simulink model "SCARA_215_ozk_test"  (R2016a)
settings: Solver=ode1  StartTime=0.0  StopTime=100  FixedStep=0.001  RelTol=1e-3
PostLoadFcn:
  | , if any(exist('dsrtsu_mdlpostloadfcn', 'file') == [2, 3, 6]), try dsrtsu_mdlpostloadfcn('Execute', bdroot); catch fprintf('Error in PostLoadFcn (dsrtsu_mdlpostloadfcn) for model "%s":\n %s\n', bdroot, lasterr); end, end,
undefined symbols (not defined in the file): sigbuilder_block
libraries: simulink x7, simulink_extras x2
settings Model: DSRTSU_INTERNAL_RTI_VER=460  DSRTSU_INTERNAL_RTI_TYPE=rti1104  Creator=k18p800a  LastModifiedBy=Piotr
settings DataIOCC: LimitDataPoints=on  SaveFormat=Array
settings OptimizationCC: BlockReduction=off  OptimizeBlockIOStorage=off  BufferReuse=off  GlobalBufferReuse=off  ExpressionFolding=off  LocalBlockOutputs=off
settings HardwareCC: ProdBitPerPointer=32  ProdLargestAtomicFloat=None  ProdEndianess=BigEndian  ProdWordSize=32  ProdHWDeviceType=Generic->Custom  TargetIntDivRoundTo=Zero  TargetEndianess=BigEndian  TargetHWDeviceType=Generic->Custom
settings ModelReferenceCC: PropagateSignalLabelsOutOfModel=off
settings RTWCC: SystemTargetFile=rti1104.tlc  MakeCommand=make_rti  TemplateMakefile=rti1104.tmf  Description=dSPACE DS1104 Hardware Platform
settings STFCustomTargetCC: ParMdlRefBuildCompliant=on  GeneratePreprocessorConditionals=Disable all  SystemTargetFile=rti1104.tlc
settings GRTTargetCC: CompOptLevelCompliant=off  ConcurrentExecutionCompliant=off  CombineOutputUpdateFcns=off  MatFileLogging=off  CPPClassGenCompliant=off  GRTInterface=on  UseToolchainInfoCompliant=off
settings ConfigComp: CovModelRefEnable=Off

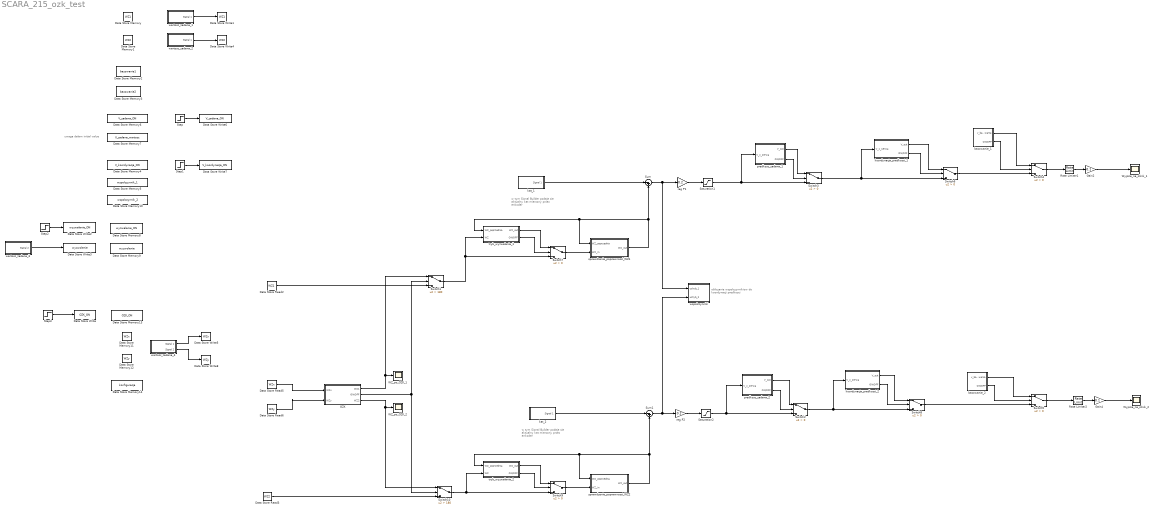
== system SCARA_215_ozk_test ==
  note: obliczanie wspolczynnikiow do
      | koordynacji predkosci
  note: w tym Signal Builder podaje
      | sie aktualny kat mierzony
      | przez enkoder
  note: w tym Signal Builder podaje
      | sie aktualny kat mierzony
      | przez enkoder
  note: uwaga dalam initial value
  Data Store Memory : DataStoreMemory  DataStoreName=WZ1  ReadBeforeWriteMsg=warning  WriteAfterWriteMsg=warning  WriteAfterReadMsg=warning  ShowAdditionalParam=off
  Data Store Memory1 : DataStoreMemory  DataStoreName=WZ2  ReadBeforeWriteMsg=warning  WriteAfterWriteMsg=warning  WriteAfterReadMsg=warning  ShowAdditionalParam=off
  Data Store Memory10 : DataStoreMemory  DataStoreName=wspolczynnik_2  ReadBeforeWriteMsg=warning  WriteAfterWriteMsg=warning  WriteAfterReadMsg=warning  ShowAdditionalParam=off
  Data Store Memory11 : DataStoreMemory  DataStoreName=WZx  ReadBeforeWriteMsg=warning  WriteAfterWriteMsg=warning  WriteAfterReadMsg=warning  ShowAdditionalParam=off
  Data Store Memory12 : DataStoreMemory  DataStoreName=WZy  ReadBeforeWriteMsg=warning  WriteAfterWriteMsg=warning  WriteAfterReadMsg=warning  ShowAdditionalParam=off
  Data Store Memory13 : DataStoreMemory  DataStoreName=OZK_ON  ReadBeforeWriteMsg=warning  WriteAfterWriteMsg=warning  WriteAfterReadMsg=warning  InitialValue=false  ShowAdditionalParam=off
  Data Store Memory14 : DataStoreMemory  DataStoreName=konfiguracja  ReadBeforeWriteMsg=warning  WriteAfterWriteMsg=warning  WriteAfterReadMsg=warning  InitialValue=false  ShowAdditionalParam=off  OutDataTypeStr=boolean
  Data Store Memory2 : DataStoreMemory  DataStoreName=bazowanie1  ReadBeforeWriteMsg=warning  WriteAfterWriteMsg=warning  WriteAfterReadMsg=warning  InitialValue=false  ShowAdditionalParam=off  OutDataTypeStr=boolean
  Data Store Memory3 : DataStoreMemory  DataStoreName=bazowanie2  ReadBeforeWriteMsg=warning  WriteAfterWriteMsg=warning  WriteAfterReadMsg=warning  InitialValue=false  ShowAdditionalParam=off  OutDataTypeStr=boolean
  Data Store Memory4 : DataStoreMemory  DataStoreName=V_koordynacja_ON  ReadBeforeWriteMsg=warning  WriteAfterWriteMsg=warning  WriteAfterReadMsg=warning  ShowAdditionalParam=off
  Data Store Memory5 : DataStoreMemory  DataStoreName=wspolczynnik_1  ReadBeforeWriteMsg=warning  WriteAfterWriteMsg=warning  WriteAfterReadMsg=warning  ShowAdditionalParam=off
  Data Store Memory6 : DataStoreMemory  DataStoreName=V_zadana_ON  ReadBeforeWriteMsg=warning  WriteAfterWriteMsg=warning  WriteAfterReadMsg=warning  ShowAdditionalParam=off
  Data Store Memory7 : DataStoreMemory  DataStoreName=V_zadana_wartosc  ReadBeforeWriteMsg=warning  WriteAfterWriteMsg=warning  WriteAfterReadMsg=warning  InitialValue=5  ShowAdditionalParam=off
  Data Store Memory8 : DataStoreMemory  DataStoreName=wyzwalanie_ON  ReadBeforeWriteMsg=warning  WriteAfterWriteMsg=warning  WriteAfterReadMsg=warning  ShowAdditionalParam=off
  Data Store Memory9 : DataStoreMemory  DataStoreName=wyzwolenie  ReadBeforeWriteMsg=warning  WriteAfterWriteMsg=warning  WriteAfterReadMsg=warning  ShowAdditionalParam=off
  Data Store Read2 : DataStoreRead  DialogController=Simulink.DDGSource  DataStoreName=WZ1
  Data Store Read3 : DataStoreRead  DialogController=Simulink.DDGSource  DataStoreName=WZ2
  Data Store Read5 : DataStoreRead  DataStoreName=WZx
  Data Store Read6 : DataStoreRead  DataStoreName=WZy
  Data Store Write : DataStoreWrite  DataStoreName=OZK_ON
  Data Store Write1 : DataStoreWrite  DataStoreName=WZ1
  Data Store Write2 : DataStoreWrite  DataStoreName=wyzwalanie_ON
  Data Store Write3 : DataStoreWrite  DataStoreName=wyzwolenie
  Data Store Write4 : DataStoreWrite  DataStoreName=WZ2
  Data Store Write5 : DataStoreWrite  DataStoreName=WZx
  Data Store Write6 : DataStoreWrite  DataStoreName=V_zadana_ON
  Data Store Write7 : DataStoreWrite  DataStoreName=V_koordynacja_ON
  Data Store Write8 : DataStoreWrite  DataStoreName=WZy
  Gain2 : Gain  Gain=0.1
  Gain4 : Gain  Gain=0.1
  OZK : Subsystem
  Rate Limiter1 : RateLimiter  RisingSlewLimit=50  FallingSlewLimit=-50  SampleTimeMode=inherited
  Rate Limiter2 : RateLimiter  RisingSlewLimit=50  FallingSlewLimit=-50  SampleTimeMode=inherited
  Saturation1 : Saturate  UpperLimit=3  LowerLimit=-3
  Saturation2 : Saturate  UpperLimit=3  LowerLimit=-3
  Step : Step  Time=50  SampleTime=0
  Step1 : Step  Time=100  SampleTime=0
  Step2 : Step  Time=100  SampleTime=0
  Step3 : Step  Time=0  SampleTime=0
  Sum : Sum  Inputs=|-+
  Sum1 : Sum  Inputs=|-+
  Switch1 : Switch  Criteria=u2 > Threshold  Threshold=180
  Switch10 : Switch  Criteria=u2 > Threshold  Threshold=180
  Switch{2..9} (8 alike) : Switch  Criteria=u2 > Threshold
  WZ_po_OZK_1 : Scope
  WZ_po_OZK_2 : Scope
  Wyjscie_na_silnik_1 : Scope
  Wyjscie_na_silnik_2 : Scope
  bazowanie_1 : Subsystem
  bazowanie_2 : Subsystem
  kat_1 : Subsystem  Tag=STV Subsys  LoadFcn=sigbuilder_block('load');  StartFcn=sigbuilder_block('start');  StopFcn=sigbuilder_block('stop');  ClipboardFcn=sigbuilder_block('clipboard');  mask(Sigbuilder block){}
      mask help: Simulink:masks:SigbuilderBlock_MD
      mask init:
      | if ~strcmp(get_param(bdroot(gcbh),'SimulationStatus'),'stopped') tuvar = sigbuilder_block('maskInit'); end
      settings: CopyFcn=sigbuilder_block('copy');  DeleteFcn=sigbuilder_block('delete');  ModelCloseFcn=sigbuilder_block('modelClose');  PreSaveFcn=sigbuilder_block('preSave');  PauseFcn=sigbuilder_block('pause');  ContinueFcn=sigbuilder_block('continue');  NameChangeFcn=sigbuilder_block('namechange');  OpenFcn=sigbuilder_block('open',[437.25 153 550.5 359.25 ]);  CloseFcn=sigbuilder_block('close');
      mask Display: plot(0, 0, 100, 100,[2, 2, 32, 32, 2], [68, 8, 8, 68, 68],[32, 2], [38, 38], [32, 19, 2],[53, 60, 44], [32, 17, 17, 2],[16, 16, 31, 31]);txt = getActiveGroup(gcbh);text(2, 100, txt,'verticalAlignment', 'top');
  kat_2 : Subsystem  Tag=STV Subsys  LoadFcn=sigbuilder_block('load');  StartFcn=sigbuilder_block('start');  StopFcn=sigbuilder_block('stop');  ClipboardFcn=sigbuilder_block('clipboard');  mask(Sigbuilder block){}
      mask help: Simulink:masks:SigbuilderBlock_MD
      mask init:
      | if ~strcmp(get_param(bdroot(gcbh),'SimulationStatus'),'stopped') tuvar = sigbuilder_block('maskInit'); end
      settings: CopyFcn=sigbuilder_block('copy');  DeleteFcn=sigbuilder_block('delete');  ModelCloseFcn=sigbuilder_block('modelClose');  PreSaveFcn=sigbuilder_block('preSave');  PauseFcn=sigbuilder_block('pause');  ContinueFcn=sigbuilder_block('continue');  NameChangeFcn=sigbuilder_block('namechange');  OpenFcn=sigbuilder_block('open',[437.25 153 550.5 359.25 ]);  CloseFcn=sigbuilder_block('close');
      mask Display: plot(0, 0, 100, 100,[2, 2, 32, 32, 2], [68, 8, 8, 68, 68],[32, 2], [38, 38], [32, 19, 2],[53, 60, 44], [32, 17, 17, 2],[16, 16, 31, 31]);txt = getActiveGroup(gcbh);text(2, 100, txt,'verticalAlignment', 'top');
  koordynacja_predkosci_1 : Subsystem
  koordynacja_predkosci_2 : Subsystem
  predkosc_zadana_1 : Subsystem
  predkosc_zadana_2 : Subsystem
  reg P1 : Gain  Gain=0.2
  reg P2 : Gain  Gain=0.2
  sprawdzenie_poprawnosci_WZ1 : Subsystem
  sprawdzenie_poprawnosci_WZ2 : Subsystem
  tryb_wyzwalania_1 : Subsystem
  tryb_wyzwalania_2 : Subsystem
  wartosc_zadana_1 : Subsystem  Tag=STV Subsys  LoadFcn=sigbuilder_block('load');  StartFcn=sigbuilder_block('start');  StopFcn=sigbuilder_block('stop');  ClipboardFcn=sigbuilder_block('clipboard');  mask(Sigbuilder block){}
      mask help: Simulink:masks:SigbuilderBlock_MD
      mask init:
      | if ~strcmp(get_param(bdroot(gcbh),'SimulationStatus'),'stopped') tuvar = sigbuilder_block('maskInit'); end
      settings: CopyFcn=sigbuilder_block('copy');  DeleteFcn=sigbuilder_block('delete');  ModelCloseFcn=sigbuilder_block('modelClose');  PreSaveFcn=sigbuilder_block('preSave');  PauseFcn=sigbuilder_block('pause');  ContinueFcn=sigbuilder_block('continue');  NameChangeFcn=sigbuilder_block('namechange');  OpenFcn=sigbuilder_block('open',[437.25 153 550.5 359.25 ]);  CloseFcn=sigbuilder_block('close');
      mask Display: plot(0, 0, 100, 100,[2, 2, 32, 32, 2], [68, 8, 8, 68, 68],[32, 2], [38, 38], [32, 19, 2],[53, 60, 44], [32, 17, 17, 2],[16, 16, 31, 31]);txt = getActiveGroup(gcbh);text(2, 100, txt,'verticalAlignment', 'top');
  wartosc_zadana_2 : Subsystem  Tag=STV Subsys  LoadFcn=sigbuilder_block('load');  StartFcn=sigbuilder_block('start');  StopFcn=sigbuilder_block('stop');  ClipboardFcn=sigbuilder_block('clipboard');  mask(Sigbuilder block){}
      mask help: Simulink:masks:SigbuilderBlock_MD
      mask init:
      | if ~strcmp(get_param(bdroot(gcbh),'SimulationStatus'),'stopped') tuvar = sigbuilder_block('maskInit'); end
      settings: CopyFcn=sigbuilder_block('copy');  DeleteFcn=sigbuilder_block('delete');  ModelCloseFcn=sigbuilder_block('modelClose');  PreSaveFcn=sigbuilder_block('preSave');  PauseFcn=sigbuilder_block('pause');  ContinueFcn=sigbuilder_block('continue');  NameChangeFcn=sigbuilder_block('namechange');  OpenFcn=sigbuilder_block('open',[437.25 153 550.5 359.25 ]);  CloseFcn=sigbuilder_block('close');
      mask Display: plot(0, 0, 100, 100,[2, 2, 32, 32, 2], [68, 8, 8, 68, 68],[32, 2], [38, 38], [32, 19, 2],[53, 60, 44], [32, 17, 17, 2],[16, 16, 31, 31]);txt = getActiveGroup(gcbh);text(2, 100, txt,'verticalAlignment', 'top');
  wartosc_zadana_3 : Subsystem  Tag=STV Subsys  LoadFcn=sigbuilder_block('load');  StartFcn=sigbuilder_block('start');  StopFcn=sigbuilder_block('stop');  ClipboardFcn=sigbuilder_block('clipboard');  mask(Sigbuilder block){}
      mask help: Simulink:masks:SigbuilderBlock_MD
      mask init:
      | if ~strcmp(get_param(bdroot(gcbh),'SimulationStatus'),'stopped') tuvar = sigbuilder_block('maskInit'); end
      settings: CopyFcn=sigbuilder_block('copy');  DeleteFcn=sigbuilder_block('delete');  ModelCloseFcn=sigbuilder_block('modelClose');  PreSaveFcn=sigbuilder_block('preSave');  PauseFcn=sigbuilder_block('pause');  ContinueFcn=sigbuilder_block('continue');  NameChangeFcn=sigbuilder_block('namechange');  OpenFcn=sigbuilder_block('open',[84.75 112.5 550.5 359.25 ]);  CloseFcn=sigbuilder_block('close');
      mask Display: plot(0, 0, 100, 100,[2, 2, 32, 32, 2], [68, 8, 8, 68, 68],[32, 2], [38, 38], [32, 19, 2],[53, 60, 44], [32, 17, 17, 2],[16, 16, 31, 31]);txt = getActiveGroup(gcbh);text(2, 100, txt,'verticalAlignment', 'top');
  wartosc_zadana_4 : Subsystem  Tag=STV Subsys  LoadFcn=sigbuilder_block('load');  StartFcn=sigbuilder_block('start');  StopFcn=sigbuilder_block('stop');  ClipboardFcn=sigbuilder_block('clipboard');  mask(Sigbuilder block){}
      mask help: Simulink:masks:SigbuilderBlock_MD
      mask init:
      | if ~strcmp(get_param(bdroot(gcbh),'SimulationStatus'),'stopped') tuvar = sigbuilder_block('maskInit'); end
      settings: CopyFcn=sigbuilder_block('copy');  DeleteFcn=sigbuilder_block('delete');  ModelCloseFcn=sigbuilder_block('modelClose');  PreSaveFcn=sigbuilder_block('preSave');  PauseFcn=sigbuilder_block('pause');  ContinueFcn=sigbuilder_block('continue');  NameChangeFcn=sigbuilder_block('namechange');  OpenFcn=sigbuilder_block('open',[437.25 153 550.5 359.25 ]);  CloseFcn=sigbuilder_block('close');
      mask Display: plot(0, 0, 100, 100,[2, 2, 32, 32, 2], [68, 8, 8, 68, 68],[32, 2], [38, 38], [32, 19, 2],[53, 60, 44], [32, 17, 17, 2],[16, 16, 31, 31]);txt = getActiveGroup(gcbh);text(2, 100, txt,'verticalAlignment', 'top');
  wspolczynniki : Subsystem
  wires:
  Rate Limiter1/1 -> Gain2/1
  Rate Limiter2/1 -> Gain4/1
  reg P1/1 -> Saturation1/1
  reg P2/1 -> Saturation2/1
  kat_1/1(Signal 1) -> Sum/1
  Gain2/1 -> Wyjscie_na_silnik_1/1
  Gain4/1 -> Wyjscie_na_silnik_2/1
  Switch4/1 -> Rate Limiter1/1
  Switch5/1 -> Rate Limiter2/1
  bazowanie_1/1(v_bazowania) -> Switch4/1
  kat_2/1(Signal 1) -> Sum1/1
  wartosc_zadana_1/1(Signal 1) -> Data Store Write1/1
  wartosc_zadana_2/1(Signal 1) -> Data Store Write4/1
  bazowanie_1/2(ON/OFF) -> Switch4/2
  bazowanie_2/2(ON/OFF) -> Switch5/2
  Sum/1 -> wspolczynniki/1(uchyb_1), reg P1/1
  Sum1/1 -> wspolczynniki/2(uchyb_2), reg P2/1
  Step/1 -> Data Store Write6/1
  Step1/1 -> Data Store Write7/1
  tryb_wyzwalania_1/2(ON/OFF) -> Switch7/2
  sprawdzenie_poprawnosci_WZ1/1(WZ_out) -> Sum/2, sprawdzenie_poprawnosci_WZ1/1(WZ_poprzednia), tryb_wyzwalania_1/1(WZ_poprzednia)
  Switch7/1 -> sprawdzenie_poprawnosci_WZ1/2(WZ_in)
  bazowanie_2/1(v_bazowania) -> Switch5/1
  tryb_wyzwalania_1/1(WZ_out) -> Switch7/1
  Saturation1/1 -> predkosc_zadana_1/1(V_z_serwa), Switch3/3
  predkosc_zadana_1/1(V_out) -> Switch3/1
  predkosc_zadana_1/2(ON/OFF) -> Switch3/2
  Switch3/1 -> Switch6/3, koordynacja_predkosci_1/1(V_z_serwa)
  Switch6/1 -> Switch4/3
  koordynacja_predkosci_1/1(V_out) -> Switch6/1
  koordynacja_predkosci_1/2(ON/OFF) -> Switch6/2
  Saturation2/1 -> predkosc_zadana_2/1(V_z_serwa), Switch2/3
  predkosc_zadana_2/1(V_out) -> Switch2/1
  predkosc_zadana_2/2(ON/OFF) -> Switch2/2
  Switch2/1 -> koordynacja_predkosci_2/1(V_z_serwa), Switch8/3
  Switch8/1 -> Switch5/3
  koordynacja_predkosci_2/1(V_out) -> Switch8/1
  koordynacja_predkosci_2/2(ON/OFF) -> Switch8/2
  tryb_wyzwalania_2/2(ON/OFF) -> Switch9/2
  sprawdzenie_poprawnosci_WZ2/1(WZ_out) -> sprawdzenie_poprawnosci_WZ2/1(WZ_poprzednia), tryb_wyzwalania_2/1(WZ_poprzednia), Sum1/2
  Switch9/1 -> sprawdzenie_poprawnosci_WZ2/2(WZ_in)
  tryb_wyzwalania_2/1(WZ_out) -> Switch9/1
  Step2/1 -> Data Store Write2/1
  wartosc_zadana_3/1(Signal 2) -> Data Store Write3/1
  Data Store Read2/1 -> Switch1/3
  Data Store Read3/1 -> Switch10/3
  Switch1/1 -> Switch7/3, tryb_wyzwalania_1/2(WZ)
  Switch10/1 -> tryb_wyzwalania_2/2(WZ), Switch9/3
  OZK/2(ON/OFF) -> Switch1/2, Switch10/2
  Data Store Read5/1 -> OZK/1(WZx)
  Data Store Read6/1 -> OZK/2("WZy ")
  OZK/3(WZ2) -> WZ_po_OZK_2/1, Switch10/1
  Step3/1 -> Data Store Write/1
  wartosc_zadana_4/1(Signal 1) -> Data Store Write5/1
  wartosc_zadana_4/2(Signal 2) -> Data Store Write8/1
  OZK/1(WZ1) -> WZ_po_OZK_1/1, Switch1/1

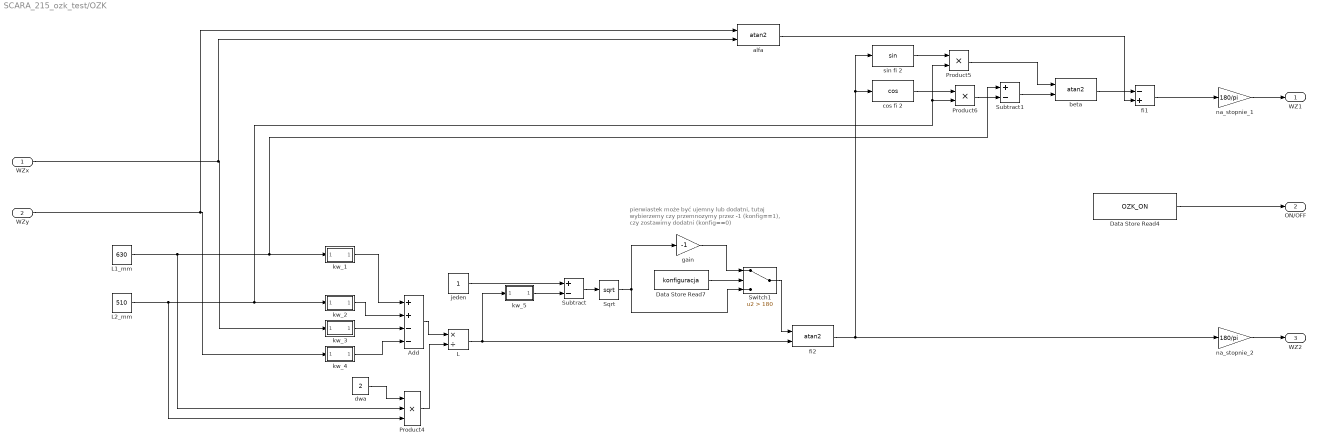
== system SCARA_215_ozk_test/OZK ==
  note: pierwiastek może być ujemny lub dodatni, tutaj wybierzemy czy przemnozymy przez -1 (konfig==1), czy zostawimy dodatni (konfig==0)
  WZx : Inport
  "WZy " : Inport  Port=2
  Add : Sum  Inputs=++--
  Data Store Read4 : DataStoreRead  DataStoreName=OZK_ON
  Data Store Read7 : DataStoreRead  DataStoreName=konfiguracja
  L : Product  Inputs=*/
  L1_mm : Constant  Value=630
  "L2_mm " : Constant  Value=510
  Product4 : Product  Inputs=3
  Product5 : Product
  Product6 : Product
  Sqrt : Sqrt  SaturateOnIntegerOverflow=on
  Subtract : Sum  Inputs=+-
  Subtract1 : Sum  Inputs=+-
  Switch1 : Switch  Criteria=u2 > Threshold  Threshold=180
  alfa : Trigonometry  Operator=atan2
  beta : Trigonometry  Operator=atan2
  "cos fi 2 " : Trigonometry  Operator=cos
  dwa : Constant  Value=2
  "fi1 " : Sum  Inputs=-+
  fi2 : Trigonometry  Operator=atan2
  gain : Gain  Gain=-1
  "jeden " : Constant
  kw_1 : Subsystem
  kw_2 : Subsystem
  kw_3 : Subsystem
  kw_4 : Subsystem
  kw_5 : Subsystem
  na_stopnie_1 : Gain  Gain=180/pi
  na_stopnie_2 : Gain  Gain=180/pi
  "sin fi 2 " : Trigonometry
  WZ1 : Outport
  ON/OFF : Outport  Port=2
  WZ2 : Outport  Port=3
  wires:
  Subtract1/1 -> beta/2
  Switch1/1 -> fi2/1
  "cos fi 2 "/1 -> Product6/1
  Product4/1 -> L/2
  Add/1 -> L/1
  Data Store Read4/1 -> ON/OFF/1
  Product6/1 -> Subtract1/2
  "WZy "/1 -> alfa/1, kw_4/1(In1)
  Sqrt/1 -> gain/1, Switch1/3
  "jeden "/1 -> Subtract/1
  Data Store Read7/1 -> Switch1/2
  L/1 -> fi2/2, kw_5/1(In1)
  "fi1 "/1 -> na_stopnie_1/1
  fi2/1 -> na_stopnie_2/1, "cos fi 2 "/1, "sin fi 2 "/1
  kw_3/1(Out1) -> Add/3
  kw_4/1(Out1) -> Add/4
  Subtract/1 -> Sqrt/1
  WZx/1 -> alfa/2, kw_3/1(In1)
  "sin fi 2 "/1 -> Product5/1
  L1_mm/1 -> Product4/2, kw_1/1(In1), Subtract1/1
  kw_2/1(Out1) -> Add/2
  Product5/1 -> beta/1
  "L2_mm "/1 -> Product4/3, kw_2/1(In1), Product5/2, Product6/2
  beta/1 -> "fi1 "/1
  kw_1/1(Out1) -> Add/1
  kw_5/1(Out1) -> Subtract/2
  gain/1 -> Switch1/1
  alfa/1 -> "fi1 "/2
  na_stopnie_1/1 -> WZ1/1
  na_stopnie_2/1 -> WZ2/1
  dwa/1 -> Product4/1

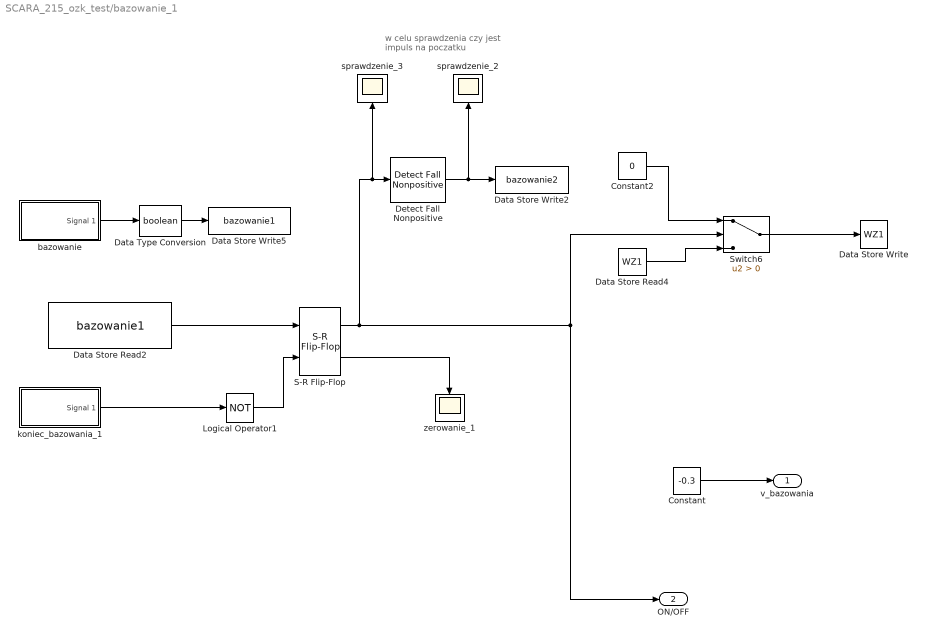
== system SCARA_215_ozk_test/bazowanie_1 ==
  note: w celu sprawdzenia czy
      | jest impuls na poczatku
  Constant : Constant  Value=-0.3
  Constant2 : Constant  Value=0
  Data Store Read2 : DataStoreRead  DataStoreName=bazowanie1
  Data Store Read4 : DataStoreRead  DialogController=Simulink.DDGSource  DataStoreName=WZ1
  Data Store Write : DataStoreWrite  DataStoreName=WZ1
  Data Store Write2 : DataStoreWrite  DataStoreName=bazowanie2
  Data Store Write5 : DataStoreWrite  DataStoreName=bazowanie1
  Data Type Conversion : DataTypeConversion  OutDataTypeStr=boolean
  Detect Fall Nonpositive : simulink/Logic and Bit Operations/Detect Fall Nonpositive  vinit=1  InputProcessing=Inherited  OutDataTypeStr=boolean
  Logical Operator1 : Logic  Operator=NOT  AllPortsSameDT=off  OutDataTypeStr=boolean
  S-R Flip-Flop : simulink_extras/Flip Flops/S-R Flip-Flop  initial_condition=0
  Switch6 : Switch  Criteria=u2 > Threshold
  bazowanie : Subsystem  Tag=STV Subsys  LoadFcn=sigbuilder_block('load');  StartFcn=sigbuilder_block('start');  StopFcn=sigbuilder_block('stop');  ClipboardFcn=sigbuilder_block('clipboard');  mask(Sigbuilder block){}
      mask help: Simulink:masks:SigbuilderBlock_MD
      mask init:
      | if ~strcmp(get_param(bdroot(gcbh),'SimulationStatus'),'stopped') tuvar = sigbuilder_block('maskInit'); end
      settings: CopyFcn=sigbuilder_block('copy');  DeleteFcn=sigbuilder_block('delete');  ModelCloseFcn=sigbuilder_block('modelClose');  PreSaveFcn=sigbuilder_block('preSave');  PauseFcn=sigbuilder_block('pause');  ContinueFcn=sigbuilder_block('continue');  NameChangeFcn=sigbuilder_block('namechange');  OpenFcn=sigbuilder_block('open',[437.25 153 550.5 359.25 ]);  CloseFcn=sigbuilder_block('close');
      mask Display: plot(0, 0, 100, 100,[2, 2, 32, 32, 2], [68, 8, 8, 68, 68],[32, 2], [38, 38], [32, 19, 2],[53, 60, 44], [32, 17, 17, 2],[16, 16, 31, 31]);txt = getActiveGroup(gcbh);text(2, 100, txt,'verticalAlignment', 'top');
  koniec_bazowania_1 : Subsystem  Tag=STV Subsys  LoadFcn=sigbuilder_block('load');  StartFcn=sigbuilder_block('start');  StopFcn=sigbuilder_block('stop');  ClipboardFcn=sigbuilder_block('clipboard');  mask(Sigbuilder block){}
      mask help: Simulink:masks:SigbuilderBlock_MD
      mask init:
      | if ~strcmp(get_param(bdroot(gcbh),'SimulationStatus'),'stopped') tuvar = sigbuilder_block('maskInit'); end
      settings: CopyFcn=sigbuilder_block('copy');  DeleteFcn=sigbuilder_block('delete');  ModelCloseFcn=sigbuilder_block('modelClose');  PreSaveFcn=sigbuilder_block('preSave');  PauseFcn=sigbuilder_block('pause');  ContinueFcn=sigbuilder_block('continue');  NameChangeFcn=sigbuilder_block('namechange');  OpenFcn=sigbuilder_block('open',[437.25 153 550.5 359.25 ]);  CloseFcn=sigbuilder_block('close');
      mask Display: plot(0, 0, 100, 100,[2, 2, 32, 32, 2], [68, 8, 8, 68, 68],[32, 2], [38, 38], [32, 19, 2],[53, 60, 44], [32, 17, 17, 2],[16, 16, 31, 31]);txt = getActiveGroup(gcbh);text(2, 100, txt,'verticalAlignment', 'top');
  sprawdzenie_2 : Scope
  sprawdzenie_3 : Scope
  zerowanie_1 : Scope
  v_bazowania : Outport
  ON/OFF : Outport  Port=2
  wires:
  koniec_bazowania_1/1(Signal 1) -> Logical Operator1/1
  Logical Operator1/1 -> S-R Flip-Flop/2
  Data Store Read4/1 -> Switch6/3
  Switch6/1 -> Data Store Write/1
  S-R Flip-Flop/2 -> zerowanie_1/1
  Data Store Read2/1 -> S-R Flip-Flop/1
  Constant2/1 -> Switch6/1
  Detect Fall Nonpositive/1 -> sprawdzenie_2/1, Data Store Write2/1
  S-R Flip-Flop/1 -> ON/OFF/1, Switch6/2, Detect Fall Nonpositive/1, sprawdzenie_3/1
  Data Type Conversion/1 -> Data Store Write5/1
  bazowanie/1(Signal 1) -> Data Type Conversion/1
  Constant/1 -> v_bazowania/1

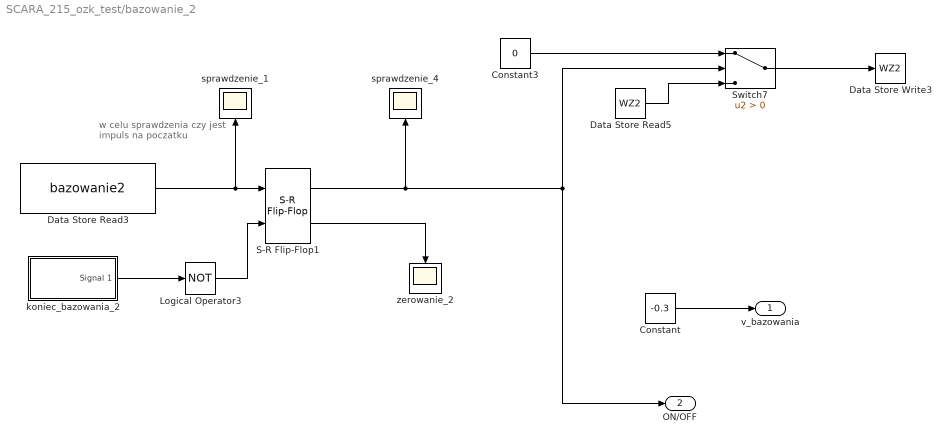
== system SCARA_215_ozk_test/bazowanie_2 ==
  note: w celu sprawdzenia czy
      | jest impuls na poczatku
  Constant : Constant  Value=-0.3
  Constant3 : Constant  Value=0
  Data Store Read3 : DataStoreRead  DataStoreName=bazowanie2
  Data Store Read5 : DataStoreRead  DialogController=Simulink.DDGSource  DataStoreName=WZ2
  Data Store Write3 : DataStoreWrite  DataStoreName=WZ2
  Logical Operator3 : Logic  Operator=NOT  AllPortsSameDT=off  OutDataTypeStr=boolean
  S-R Flip-Flop1 : simulink_extras/Flip Flops/S-R Flip-Flop  initial_condition=0
  Switch7 : Switch  Criteria=u2 > Threshold
  "koniec_bazowania_2 " : Subsystem  Tag=STV Subsys  LoadFcn=sigbuilder_block('load');  StartFcn=sigbuilder_block('start');  StopFcn=sigbuilder_block('stop');  ClipboardFcn=sigbuilder_block('clipboard');  mask(Sigbuilder block){}
      mask help: Simulink:masks:SigbuilderBlock_MD
      mask init:
      | if ~strcmp(get_param(bdroot(gcbh),'SimulationStatus'),'stopped') tuvar = sigbuilder_block('maskInit'); end
      settings: CopyFcn=sigbuilder_block('copy');  DeleteFcn=sigbuilder_block('delete');  ModelCloseFcn=sigbuilder_block('modelClose');  PreSaveFcn=sigbuilder_block('preSave');  PauseFcn=sigbuilder_block('pause');  ContinueFcn=sigbuilder_block('continue');  NameChangeFcn=sigbuilder_block('namechange');  OpenFcn=sigbuilder_block('open',[437.25 153 550.5 359.25 ]);  CloseFcn=sigbuilder_block('close');
      mask Display: plot(0, 0, 100, 100,[2, 2, 32, 32, 2], [68, 8, 8, 68, 68],[32, 2], [38, 38], [32, 19, 2],[53, 60, 44], [32, 17, 17, 2],[16, 16, 31, 31]);txt = getActiveGroup(gcbh);text(2, 100, txt,'verticalAlignment', 'top');
  sprawdzenie_1 : Scope
  sprawdzenie_4 : Scope
  zerowanie_2 : Scope
  v_bazowania : Outport
  ON/OFF : Outport  Port=2
  wires:
  S-R Flip-Flop1/2 -> zerowanie_2/1
  Data Store Read3/1 -> sprawdzenie_1/1, S-R Flip-Flop1/1
  Logical Operator3/1 -> S-R Flip-Flop1/2
  Switch7/1 -> Data Store Write3/1
  "koniec_bazowania_2 "/1(Signal 1) -> Logical Operator3/1
  Constant3/1 -> Switch7/1
  Data Store Read5/1 -> Switch7/3
  S-R Flip-Flop1/1 -> sprawdzenie_4/1, ON/OFF/1, Switch7/2
  Constant/1 -> v_bazowania/1

== system SCARA_215_ozk_test/kat_1 ==
  Demux : Demux  Tag=STV Demux  Outputs=1
  FromWs : FromWorkspace  Tag=STV FromWs  VariableName=tuvar  SampleTime=0
      SigBuilderData=|
      | common.afterFinalStr = 'Extrapolate'
      | common.sampleTime = 0
      | dataSet.timeRange = [0 100]
      | dataSet.name = 'Group 1'
      | sbobj.Groups.Name = 'Group 1'
      | sbobj.Groups.Signals.Name = 'Signal 1'
      | sbobj.Groups.Signals.XData = [0 4 6 100]
      | sbobj.Groups.Signals.YData = [0 0 0 0]
      | sbobj.Groups.TimeRange = [0 100]
  Signal 1 : Outport  Tag=STV Outport
  wires:
  Demux/1 -> Signal 1/1
  FromWs/1 -> Demux/1

== system SCARA_215_ozk_test/kat_2 ==
  Demux : Demux  Tag=STV Demux  Outputs=1
  FromWs : FromWorkspace  Tag=STV FromWs  VariableName=tuvar  SampleTime=0
      SigBuilderData=|
      | common.afterFinalStr = 'Extrapolate'
      | common.sampleTime = 0
      | dataSet.timeRange = [0 100]
      | dataSet.name = 'Group 1'
      | sbobj.Groups.Name = 'Group 1'
      | sbobj.Groups.Signals.Name = 'Signal 1'
      | sbobj.Groups.Signals.XData = [0 4 6 100]
      | sbobj.Groups.Signals.YData = [0 0 0 0]
      | sbobj.Groups.TimeRange = [0 100]
  Signal 1 : Outport  Tag=STV Outport
  wires:
  Demux/1 -> Signal 1/1
  FromWs/1 -> Demux/1

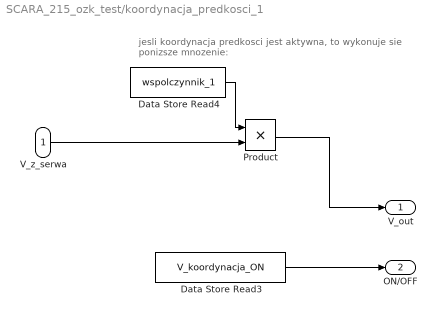
== system SCARA_215_ozk_test/koordynacja_predkosci_1 ==
  note: jesli koordynacja predkosci jest aktywna, to wykonuje sie ponizsze mnozenie:
  V_z_serwa : Inport
  Data Store Read3 : DataStoreRead  DataStoreName=V_koordynacja_ON
  Data Store Read4 : DataStoreRead  DataStoreName=wspolczynnik_1
  Product : Product
  V_out : Outport
  ON/OFF : Outport  Port=2
  wires:
  Data Store Read4/1 -> Product/1
  Data Store Read3/1 -> ON/OFF/1
  Product/1 -> V_out/1
  V_z_serwa/1 -> Product/2

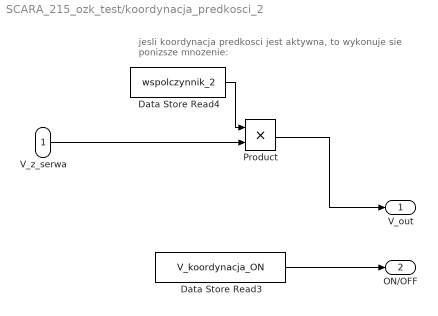
== system SCARA_215_ozk_test/koordynacja_predkosci_2 ==
  note: jesli koordynacja predkosci jest aktywna, to wykonuje sie ponizsze mnozenie:
  V_z_serwa : Inport
  Data Store Read3 : DataStoreRead  DataStoreName=V_koordynacja_ON
  Data Store Read4 : DataStoreRead  DataStoreName=wspolczynnik_2
  Product : Product
  V_out : Outport
  ON/OFF : Outport  Port=2
  wires:
  Data Store Read4/1 -> Product/1
  Data Store Read3/1 -> ON/OFF/1
  Product/1 -> V_out/1
  V_z_serwa/1 -> Product/2

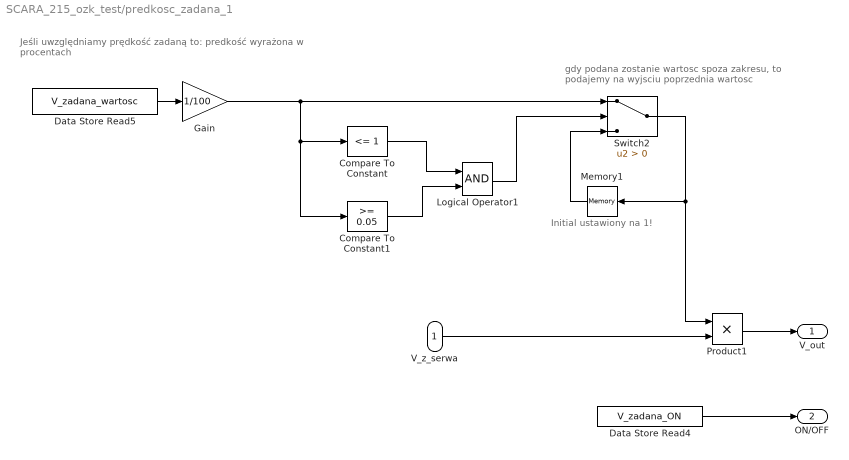
== system SCARA_215_ozk_test/predkosc_zadana_1 ==
  note: Initial ustawiony na 1!
  note: gdy podana zostanie wartosc spoza zakresu,
      | to podajemy na wyjsciu poprzednia wartosc
  note: Jeśli uwzględniamy prędkość zadaną to: predkość wyrażona w procentach
  V_z_serwa : Inport
  Compare To Constant : simulink/Logic and Bit Operations/Compare To Constant  relop=<=  const=1  OutDataTypeStr=boolean
  Compare To Constant1 : simulink/Logic and Bit Operations/Compare To Constant  relop=>=  const=0.05  OutDataTypeStr=boolean
  Data Store Read4 : DataStoreRead  DataStoreName=V_zadana_ON
  Data Store Read5 : DataStoreRead  DataStoreName=V_zadana_wartosc
  Gain : Gain  Gain=1/100
  Logical Operator1 : Logic  AllPortsSameDT=off  OutDataTypeStr=boolean
  Memory1 : Memory  X0=1
  Product1 : Product
  Switch2 : Switch  Criteria=u2 > Threshold
  V_out : Outport
  ON/OFF : Outport  Port=2
  wires:
  V_z_serwa/1 -> Product1/2
  Compare To Constant/1 -> Logical Operator1/1
  Compare To Constant1/1 -> Logical Operator1/2
  Data Store Read4/1 -> ON/OFF/1
  Data Store Read5/1 -> Gain/1
  Gain/1 -> Switch2/1, Compare To Constant1/1, Compare To Constant/1
  Product1/1 -> V_out/1
  Memory1/1 -> Switch2/3
  Logical Operator1/1 -> Switch2/2
  Switch2/1 -> Product1/1, Memory1/1

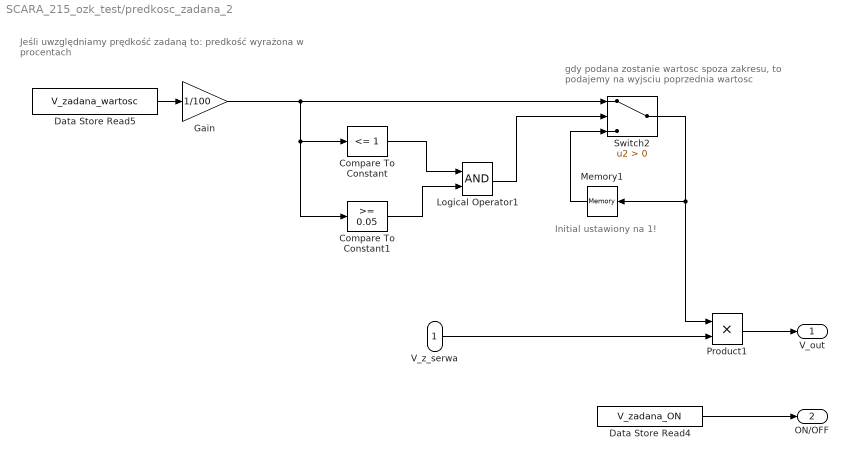
== system SCARA_215_ozk_test/predkosc_zadana_2 ==
  note: Initial ustawiony na 1!
  note: gdy podana zostanie wartosc spoza zakresu,
      | to podajemy na wyjsciu poprzednia wartosc
  note: Jeśli uwzględniamy prędkość zadaną to: predkość wyrażona w procentach
  V_z_serwa : Inport
  Compare To Constant : simulink/Logic and Bit Operations/Compare To Constant  relop=<=  const=1  OutDataTypeStr=boolean
  Compare To Constant1 : simulink/Logic and Bit Operations/Compare To Constant  relop=>=  const=0.05  OutDataTypeStr=boolean
  Data Store Read4 : DataStoreRead  DataStoreName=V_zadana_ON
  Data Store Read5 : DataStoreRead  DataStoreName=V_zadana_wartosc
  Gain : Gain  Gain=1/100
  Logical Operator1 : Logic  AllPortsSameDT=off  OutDataTypeStr=boolean
  Memory1 : Memory  X0=1
  Product1 : Product
  Switch2 : Switch  Criteria=u2 > Threshold
  V_out : Outport
  ON/OFF : Outport  Port=2
  wires:
  V_z_serwa/1 -> Product1/2
  Compare To Constant/1 -> Logical Operator1/1
  Compare To Constant1/1 -> Logical Operator1/2
  Data Store Read4/1 -> ON/OFF/1
  Data Store Read5/1 -> Gain/1
  Gain/1 -> Switch2/1, Compare To Constant1/1, Compare To Constant/1
  Product1/1 -> V_out/1
  Memory1/1 -> Switch2/3
  Logical Operator1/1 -> Switch2/2
  Switch2/1 -> Product1/1, Memory1/1

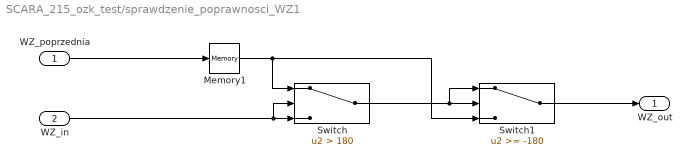
== system SCARA_215_ozk_test/sprawdzenie_poprawnosci_WZ1 ==
  WZ_poprzednia : Inport
  WZ_in : Inport  Port=2
  Memory1 : Memory
  Switch : Switch  Criteria=u2 > Threshold  Threshold=180
  Switch1 : Switch  Threshold=-180
  WZ_out : Outport
  wires:
  Switch/1 -> Switch1/1, Switch1/2
  Memory1/1 -> Switch1/3, Switch/1
  Switch1/1 -> WZ_out/1
  WZ_poprzednia/1 -> Memory1/1
  WZ_in/1 -> Switch/2, Switch/3

== system SCARA_215_ozk_test/sprawdzenie_poprawnosci_WZ2 ==
  WZ_poprzednia : Inport
  WZ_in : Inport  Port=2
  Memory1 : Memory
  Switch : Switch  Criteria=u2 > Threshold  Threshold=180
  Switch1 : Switch  Threshold=-180
  WZ_out : Outport
  wires:
  Switch/1 -> Switch1/1, Switch1/2
  Memory1/1 -> Switch1/3, Switch/1
  Switch1/1 -> WZ_out/1
  WZ_poprzednia/1 -> Memory1/1
  WZ_in/1 -> Switch/2, Switch/3

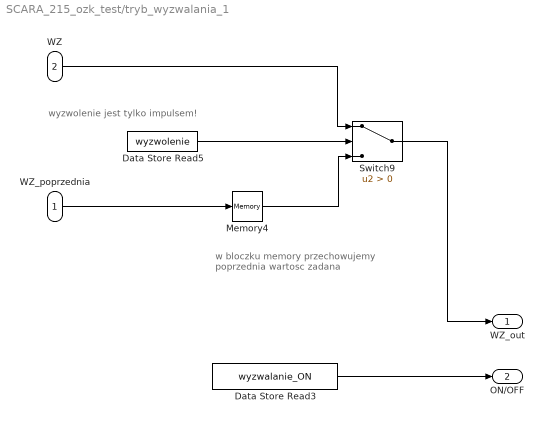
== system SCARA_215_ozk_test/tryb_wyzwalania_1 ==
  note: wyzwolenie jest tylko impulsem!
  note: w bloczku memory przechowujemy
      | poprzednia wartosc zadana
  WZ_poprzednia : Inport
  WZ : Inport  Port=2
  Data Store Read3 : DataStoreRead  DataStoreName=wyzwalanie_ON
  Data Store Read5 : DataStoreRead  DialogController=Simulink.DDGSource  DataStoreName=wyzwolenie
  Memory4 : Memory
  Switch9 : Switch  Criteria=u2 > Threshold
  WZ_out : Outport
  ON/OFF : Outport  Port=2
  wires:
  Data Store Read5/1 -> Switch9/2
  Switch9/1 -> WZ_out/1
  Memory4/1 -> Switch9/3
  WZ/1 -> Switch9/1
  WZ_poprzednia/1 -> Memory4/1
  Data Store Read3/1 -> ON/OFF/1

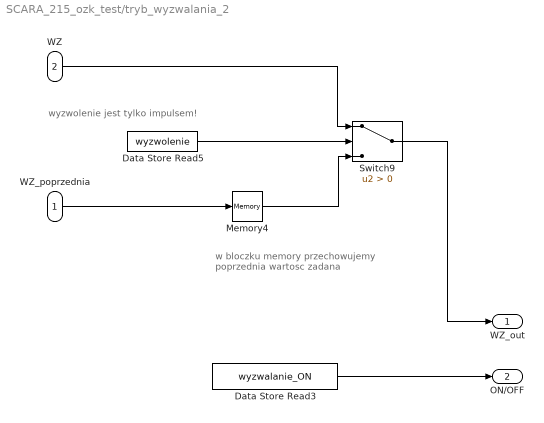
== system SCARA_215_ozk_test/tryb_wyzwalania_2 ==
  note: wyzwolenie jest tylko impulsem!
  note: w bloczku memory przechowujemy
      | poprzednia wartosc zadana
  WZ_poprzednia : Inport
  WZ : Inport  Port=2
  Data Store Read3 : DataStoreRead  DataStoreName=wyzwalanie_ON
  Data Store Read5 : DataStoreRead  DialogController=Simulink.DDGSource  DataStoreName=wyzwolenie
  Memory4 : Memory
  Switch9 : Switch  Criteria=u2 > Threshold
  WZ_out : Outport
  ON/OFF : Outport  Port=2
  wires:
  Data Store Read5/1 -> Switch9/2
  Switch9/1 -> WZ_out/1
  Memory4/1 -> Switch9/3
  WZ/1 -> Switch9/1
  WZ_poprzednia/1 -> Memory4/1
  Data Store Read3/1 -> ON/OFF/1

== system SCARA_215_ozk_test/wartosc_zadana_1 ==
  Demux : Demux  Tag=STV Demux  Outputs=1
  FromWs : FromWorkspace  Tag=STV FromWs  VariableName=tuvar  SampleTime=0
      SigBuilderData=|
      | common.afterFinalStr = 'Extrapolate'
      | common.sampleTime = 0
      | dataSet.timeRange = [0 100]
      | dataSet.name = 'Group 1'
      | sbobj.Groups.Name = 'Group 1'
      | sbobj.Groups.Signals.Name = 'Signal 1'
      | sbobj.Groups.Signals.XData = [0 5 5 50 50 100]
      | sbobj.Groups.Signals.YData = [0 0 190 190 0 0]
      | sbobj.Groups.TimeRange = [0 100]
  Signal 1 : Outport  Tag=STV Outport
  wires:
  Demux/1 -> Signal 1/1
  FromWs/1 -> Demux/1

== system SCARA_215_ozk_test/wartosc_zadana_2 ==
  Demux : Demux  Tag=STV Demux  Outputs=1
  FromWs : FromWorkspace  Tag=STV FromWs  VariableName=tuvar  SampleTime=0
      SigBuilderData=|
      | common.afterFinalStr = 'Extrapolate'
      | common.sampleTime = 0
      | dataSet.timeRange = [0 100]
      | dataSet.name = 'Group 1'
      | sbobj.Groups.Name = 'Group 1'
      | sbobj.Groups.Signals.Name = 'Signal 1'
      | sbobj.Groups.Signals.XData = [0 5 5 50 50 100]
      | sbobj.Groups.Signals.YData = [0 0 45 45 0 0]
      | sbobj.Groups.TimeRange = [0 100]
  Signal 1 : Outport  Tag=STV Outport
  wires:
  Demux/1 -> Signal 1/1
  FromWs/1 -> Demux/1

== system SCARA_215_ozk_test/wartosc_zadana_3 ==
  Demux : Demux  Tag=STV Demux  Outputs=1
  FromWs : FromWorkspace  Tag=STV FromWs  VariableName=tuvar  SampleTime=0
      SigBuilderData=|
      | common.afterFinalStr = 'Extrapolate'
      | common.sampleTime = 0
      | dataSet(1).timeRange = [0 100]
      | dataSet(1).name = 'Group 1'
      | dataSet(2).timeRange = [0 100]
      | dataSet(2).name = 'Group 2'
      | sbobj.Groups(1).Name = 'Group 1'
      | sbobj.Groups(1).Signals.Name = 'Signal 2'
      | sbobj.Groups(1).Signals.XData = [0 0 12.5 12.5 25 25 37.5 37.5 50 50 62.5 62.5 75 75 87.5 87.5 100 100]
      | sbobj.Groups(1).Signals.YData = [-1 1 1 -1 -1 1 1 -1 -1 1 1 -1 -1 1 1 -1 -1 1]
      | sbobj.Groups(1).TimeRange = [0 100]
      | sbobj.Groups(2).Name = 'Group 2'
      | sbobj.Groups(2).Signals.Name = 'Signal 2'
      | sbobj.Groups(2).Signals.XData = [0 12.5 25 25 25.4 25.4 62.2 62.2 62.5 62.5 85.8 85.8 87.5 87.5 100]
      | sbobj.Groups(2).Signals.YData = [0 0 0 1 1 0 0 1 1 0 0 1 1 0 0]
      | sbobj.Groups(2).TimeRange = [0 100]
  Signal 2 : Outport  Tag=STV Outport
  wires:
  FromWs/1 -> Demux/1
  Demux/1 -> Signal 2/1

== system SCARA_215_ozk_test/wartosc_zadana_4 ==
  Demux : Demux  Tag=STV Demux  Outputs=2
  FromWs : FromWorkspace  Tag=STV FromWs  VariableName=tuvar  SampleTime=0
      SigBuilderData=|
      | common.afterFinalStr = 'Extrapolate'
      | common.sampleTime = 0
      | dataSet(1).timeRange = [0 100]
      | dataSet(1).name = '135_180'
      | dataSet(2).timeRange = [0 100]
      | dataSet(2).name = '-135_180'
      | dataSet(3).timeRange = [0 100]
      | dataSet(3).name = '45_180'
      | dataSet(4).timeRange = [0 100]
      | dataSet(4).name = '-45_180'
      | sbobj.Groups(1).Name = '135_180'
      | sbobj.Groups(1).Signals(1).Name = 'Signal 1'
      | sbobj.Groups(1).Signals(1).XData = [0 10 10 50 50 100]
      | sbobj.Groups(1).Signals(1).YData = [0 0 -806.101 -806.101 0 0]
      | sbobj.Groups(1).Signals(2).Name = 'Signal 2'
      | sbobj.Groups(1).Signals(2).XData = [0 10 10 50 50 100]
      | sbobj.Groups(1).Signals(2).YData = [0 0 806.101 806.101 0 0]
      | sbobj.Groups(1).TimeRange = [0 100]
      | sbobj.Groups(2).Name = '-135_180'
      | sbobj.Groups(2).Signals(1).Name = 'Signal 1'
      | sbobj.Groups(2).Signals(1).XData = [0 10 10 50 50 100]
      | sbobj.Groups(2).Signals(1).YData = [0 0 -806.101 -806.101 0 0]
      | sbobj.Groups(2).Signals(2).Name = 'Signal 2'
      | sbobj.Groups(2).Signals(2).XData = [0 10 10 50 50 100]
      | sbobj.Groups(2).Signals(2).YData = [0 0 -806.101 -806.101 0 0]
      | sbobj.Groups(2).TimeRange = [0 100]
      | sbobj.Groups(3).Name = '45_180'
      | sbobj.Groups(3).Signals(1).Name = 'Signal 1'
      | sbobj.Groups(3).Signals(1).XData = [0 10 10 50 50 100]
      | sbobj.Groups(3).Signals(1).YData = [0 0 806.101 806.101 0 0]
      | sbobj.Groups(3).Signals(2).Name = 'Signal 2'
      | sbobj.Groups(3).Signals(2).XData = [0 10 10 50 50 100]
      | sbobj.Groups(3).Signals(2).YData = [0 0 806.101 806.101 0 0]
      | sbobj.Groups(3).TimeRange = [0 100]
      | sbobj.Groups(4).Name = '-45_180'
      | sbobj.Groups(4).Signals(1).Name = 'Signal 1'
      | sbobj.Groups(4).Signals(1).XData = [0 10 10 50 50 100]
      | sbobj.Groups(4).Signals(1).YData = [0 0 806.101 806.101 0 0]
      | sbobj.Groups(4).Signals(2).Name = 'Signal 2'
      | sbobj.Groups(4).Signals(2).XData = [0 10 10 50 50 100]
      | sbobj.Groups(4).Signals(2).YData = [0 0 -806.101 -806.101 0 0]
      | sbobj.Groups(4).TimeRange = [0 100]
  Signal 1 : Outport  Tag=STV Outport
  Signal 2 : Outport  Tag=STV Outport  Port=2
  wires:
  Demux/1 -> Signal 1/1
  FromWs/1 -> Demux/1
  Demux/2 -> Signal 2/1

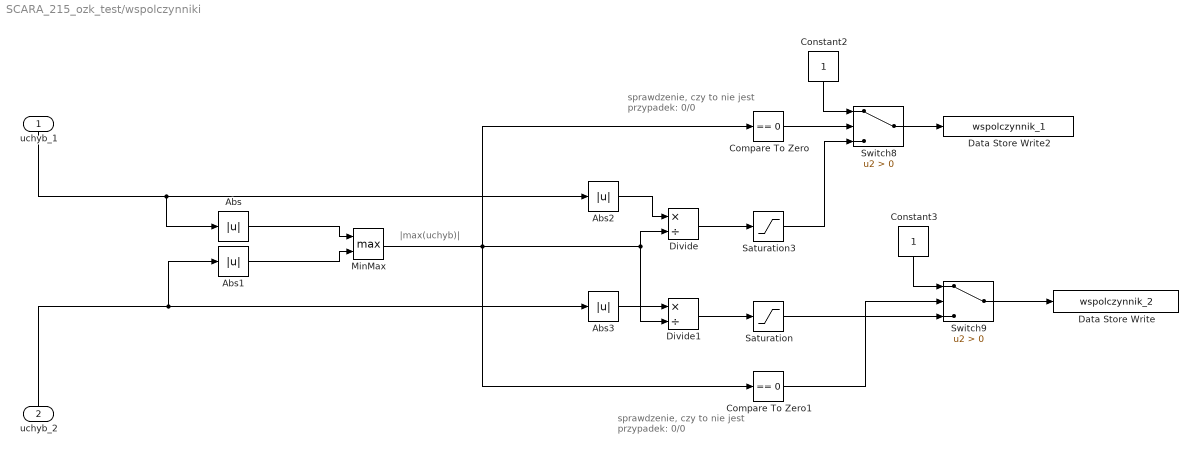
== system SCARA_215_ozk_test/wspolczynniki ==
  note: sprawdzenie, czy to nie
      | jest przypadek: 0/0
  note: sprawdzenie, czy to nie
      | jest przypadek: 0/0
  note: |max(uchyb)|
  uchyb_1 : Inport
  uchyb_2 : Inport  Port=2
  Abs{,1..3} (4 alike) : Abs
  Compare To Zero : simulink/Logic and Bit Operations/Compare To Zero  relop===  OutDataTypeStr=boolean
  Compare To Zero1 : simulink/Logic and Bit Operations/Compare To Zero  relop===  OutDataTypeStr=boolean
  Constant2 : Constant
  Constant3 : Constant
  Data Store Write : DataStoreWrite  DataStoreName=wspolczynnik_2
  Data Store Write2 : DataStoreWrite  DataStoreName=wspolczynnik_1
  Divide : Product  Inputs=*/
  Divide1 : Product  Inputs=*/
  MinMax : MinMax  Function=max  Inputs=2
  Saturation : Saturate  UpperLimit=1  LowerLimit=0.05
  Saturation3 : Saturate  UpperLimit=1  LowerLimit=0.05
  Switch8 : Switch  Criteria=u2 > Threshold
  Switch9 : Switch  Criteria=u2 > Threshold
  wires:
  Compare To Zero1/1 -> Switch9/2
  Constant3/1 -> Switch9/1
  Constant2/1 -> Switch8/1
  Switch9/1 -> Data Store Write/1
  Compare To Zero/1 -> Switch8/2
  Abs2/1 -> Divide/1
  Abs3/1 -> Divide1/1
  MinMax/1 -> Compare To Zero1/1, Compare To Zero/1, Divide1/2, Divide/2
  Abs/1 -> MinMax/1
  Abs1/1 -> MinMax/2
  Divide1/1 -> Saturation/1
  Saturation/1 -> Switch9/3
  Divide/1 -> Saturation3/1
  Saturation3/1 -> Switch8/3
  uchyb_1/1 -> Abs/1, Abs2/1
  uchyb_2/1 -> Abs1/1, Abs3/1
  Switch8/1 -> Data Store Write2/1

== system SCARA_215_ozk_test/OZK/kw_1 ==
  In1 : Inport
  Product : Product
  Out1 : Outport
  wires:
  Product/1 -> Out1/1
  In1/1 -> Product/2, Product/1

== system SCARA_215_ozk_test/OZK/kw_2 ==
  In1 : Inport
  Product : Product
  Out1 : Outport
  wires:
  Product/1 -> Out1/1
  In1/1 -> Product/2, Product/1

== system SCARA_215_ozk_test/OZK/kw_3 ==
  In1 : Inport
  Product : Product
  Out1 : Outport
  wires:
  Product/1 -> Out1/1
  In1/1 -> Product/2, Product/1

== system SCARA_215_ozk_test/OZK/kw_4 ==
  In1 : Inport
  Product : Product
  Out1 : Outport
  wires:
  Product/1 -> Out1/1
  In1/1 -> Product/2, Product/1

== system SCARA_215_ozk_test/OZK/kw_5 ==
  In1 : Inport
  Product : Product
  Out1 : Outport
  wires:
  Product/1 -> Out1/1
  In1/1 -> Product/2, Product/1

== system SCARA_215_ozk_test/bazowanie_1/bazowanie ==
  Demux : Demux  Tag=STV Demux  Outputs=1
  FromWs : FromWorkspace  Tag=STV FromWs  VariableName=tuvar  SampleTime=0
      SigBuilderData=|
      | common.afterFinalStr = 'Extrapolate'
      | common.sampleTime = 0
      | dataSet.timeRange = [0 100]
      | dataSet.name = 'Group 1'
      | sbobj.Groups.Name = 'Group 1'
      | sbobj.Groups.Signals.Name = 'Signal 1'
      | sbobj.Groups.Signals.XData = [0 2.6 22.6 100]
      | sbobj.Groups.Signals.YData = [0 0 0 0]
      | sbobj.Groups.TimeRange = [0 100]
  Signal 1 : Outport  Tag=STV Outport
  wires:
  Demux/1 -> Signal 1/1
  FromWs/1 -> Demux/1

== system SCARA_215_ozk_test/bazowanie_1/koniec_bazowania_1 ==
  Demux : Demux  Tag=STV Demux  Outputs=1
  FromWs : FromWorkspace  Tag=STV FromWs  VariableName=tuvar  SampleTime=0
      SigBuilderData=|
      | common.afterFinalStr = 'Extrapolate'
      | common.sampleTime = 0
      | dataSet.timeRange = [0 100]
      | dataSet.name = 'Group 1'
      | sbobj.Groups.Name = 'Group 1'
      | sbobj.Groups.Signals.Name = 'Signal 1'
      | sbobj.Groups.Signals.XData = [0 10 10 12 12 100]
      | sbobj.Groups.Signals.YData = [1 1 0 0 1 1]
      | sbobj.Groups.TimeRange = [0 100]
  Signal 1 : Outport  Tag=STV Outport
  wires:
  Demux/1 -> Signal 1/1
  FromWs/1 -> Demux/1

== system SCARA_215_ozk_test/bazowanie_2/koniec_bazowania_2  ==
  Demux : Demux  Tag=STV Demux  Outputs=1
  FromWs : FromWorkspace  Tag=STV FromWs  VariableName=tuvar  SampleTime=0
      SigBuilderData=|
      | common.afterFinalStr = 'Extrapolate'
      | common.sampleTime = 0
      | dataSet.timeRange = [0 100]
      | dataSet.name = 'Group 1'
      | sbobj.Groups.Name = 'Group 1'
      | sbobj.Groups.Signals.Name = 'Signal 1'
      | sbobj.Groups.Signals.XData = [0 50.6 50.6 52.6 52.6 100]
      | sbobj.Groups.Signals.YData = [1 1 0 0 1 1]
      | sbobj.Groups.TimeRange = [0 100]
  Signal 1 : Outport  Tag=STV Outport
  wires:
  Demux/1 -> Signal 1/1
  FromWs/1 -> Demux/1
